simulink model "gm_uz_pmsm_model_3ph_dq_vnl"  (R2021b)
settings: Solver=FixedStepAuto  StartTime=0.0  StopTime=0.5  RelTol=1e-3
PreLoadFcn:
  | uz_pmsm_model_init_parameter
undefined symbols (not defined in the file or in its folder): friction_coefficient, inertia, k_i_d, k_p_d, k_p_q, L_d, L_q, polepair, psi_pm, R_1, setpoint_step, simulate_mechanical, simulate_open_loop, static_friction_torque, ts, ts_regler
libraries: hdlmdlgenlib x69, dspsigops x18, simulink x12, slpidlib x2
(part 2 of 2)

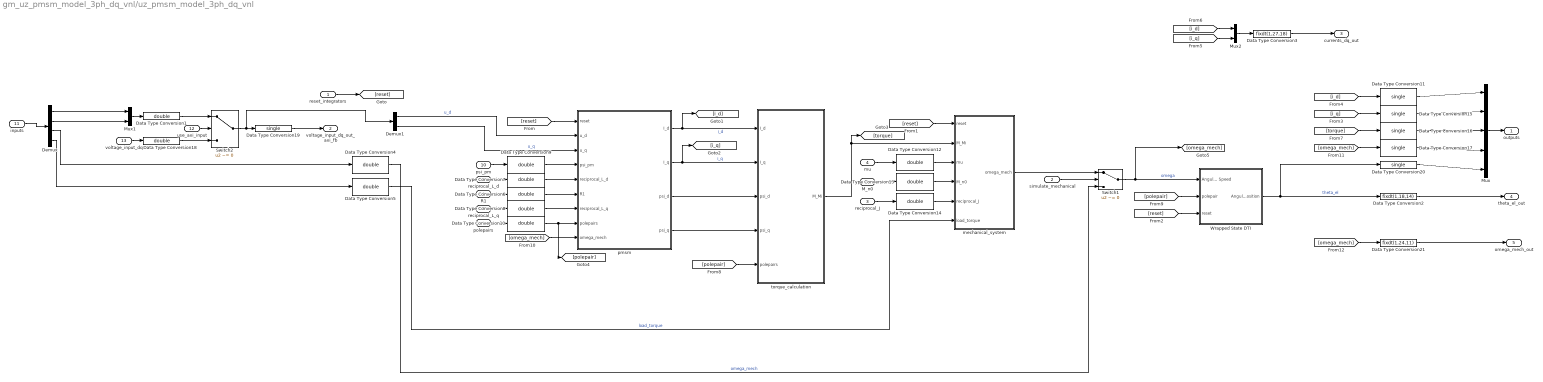
== system gm_uz_pmsm_model_3ph_dq_vnl/uz_pmsm_model_3ph_dq_vnl ==
  reset_integrators : Inport
  simulate_mechanical : Inport  Port=2
  reciprocal_J : Inport  Port=3
  mu : Inport  Port=4
  M_n0 : Inport  Port=5
  reciprocal_L_d : Inport  Port=6
  reciprocal_L_q : Inport  Port=7
  R1 : Inport  Port=8
  polepairs : Inport  Port=9
  psi_pm : Inport  Port=10
  inputs : Inport  Port=11
  use_axi_input : Inport  Port=12
  voltage_input_dq : Inport  Port=13
  Data Type Conversion{1,4..10,12..14,18} (12 alike) : DataTypeConversion  OutDataTypeStr=double  RndMeth=Nearest
  Data Type Conversion{11,15..17,19..20} (6 alike) : DataTypeConversion  OutDataTypeStr=single  RndMeth=Nearest
  Data Type Conversion2 : DataTypeConversion  OutDataTypeStr=fixdt(1,18,14)  RndMeth=Nearest
  Data Type Conversion21 : DataTypeConversion  OutDataTypeStr=fixdt(1,24,11)  RndMeth=Nearest
  Data Type Conversion3 : DataTypeConversion  OutDataTypeStr=fixdt(1,27,18)  RndMeth=Nearest
  Demux : Demux
  Demux1 : Demux  Outputs=2
  Mux : Mux  Inputs=5
  Mux1 : Mux  Inputs=2
  Mux2 : Mux  Inputs=2
  Switch1 : Switch  Criteria=u2 ~= 0
  Switch2 : Switch  Criteria=u2 ~= 0
  Wrapped State DTI : Subsystem
  mechanical_system : Subsystem
  pmsm : Subsystem
  torque_calculation : Subsystem
  outputs : Outport
  voltage_input_dq_out_axi_fb : Outport  Port=2
  currents_dq_out : Outport  Port=3
  theta_el_out : Outport  Port=4
  omega_mech_out : Outport  Port=5
  wires:
  [omega_mech] -> Data Type Conversion21/1
  Data Type Conversion21/1 -> omega_mech_out/1
  Data Type Conversion18/1 -> Switch2/3
  Data Type Conversion1/1 -> Switch2/1
  [omega_mech] -> Data Type Conversion17/1
  [omega_mech] -> pmsm/9(omega_mech)
  [polepair] -> Wrapped State DTI/2(polepair)
  [polepair] -> torque_calculation/5(polepairs)
  [torque] -> Data Type Conversion16/1
  [i_q] -> Mux2/2
  [i_d] -> Mux2/1
  [i_d] -> Data Type Conversion11/1
  [i_q] -> Data Type Conversion15/1
  pmsm/1(I_d) -> [i_d], torque_calculation/1(I_d)  "i_d"
  [reset] -> Wrapped State DTI/3(reset)
  [reset] -> mechanical_system/1(reset)
  [reset] -> pmsm/1(reset)
  reset_integrators/1 -> [reset]
  Data Type Conversion20/1 -> Mux/5
  Data Type Conversion2/1 -> theta_el_out/1
  Wrapped State DTI/1(Angular Position) -> Data Type Conversion20/1, Data Type Conversion2/1  "theta_el"
  Mux2/1 -> Data Type Conversion3/1
  Data Type Conversion3/1 -> currents_dq_out/1
  Demux/2 -> Mux1/2
  Demux/1 -> Mux1/1
  use_axi_input/1 -> Switch2/2
  Mux1/1 -> Data Type Conversion1/1
  Switch2/1 -> Data Type Conversion19/1, Demux1/1
  voltage_input_dq/1 -> Data Type Conversion18/1
  Data Type Conversion19/1 -> voltage_input_dq_out_axi_fb/1
  Mux/1 -> outputs/1
  inputs/1 -> Demux/1
  Demux/4 -> Data Type Conversion5/1
  Demux/3 -> Data Type Conversion4/1
  Data Type Conversion11/1 -> Mux/1
  Data Type Conversion15/1 -> Mux/2
  Data Type Conversion16/1 -> Mux/3
  Data Type Conversion17/1 -> Mux/4
  pmsm/2(I_q) -> torque_calculation/2(I_q), [i_q]  "i_q"
  mechanical_system/1(omega_mech) -> Switch1/1
  Demux1/2 -> pmsm/3(u_q)  "u_q"
  polepairs/1 -> Data Type Conversion10/1
  reciprocal_L_q/1 -> Data Type Conversion8/1
  Data Type Conversion8/1 -> pmsm/7(reciprocal_L_q)
  reciprocal_L_d/1 -> Data Type Conversion7/1
  Data Type Conversion13/1 -> mechanical_system/4(M_n0)
  psi_pm/1 -> Data Type Conversion9/1
  mu/1 -> Data Type Conversion12/1
  torque_calculation/1(M_Mi) -> mechanical_system/2(M_Mi), [torque]
  Data Type Conversion14/1 -> mechanical_system/5(reciprocal_J)
  M_n0/1 -> Data Type Conversion13/1
  simulate_mechanical/1 -> Switch1/2
  Data Type Conversion12/1 -> mechanical_system/3(mu)
  Demux1/1 -> pmsm/2(u_d)  "u_d"
  Data Type Conversion10/1 -> pmsm/8(polepairs), [polepair]
  pmsm/4(psi_q) -> torque_calculation/4(psi_q)
  Data Type Conversion6/1 -> pmsm/6(R1)
  R1/1 -> Data Type Conversion6/1
  Data Type Conversion9/1 -> pmsm/4(psi_pm)
  Switch1/1 -> [omega_mech], Wrapped State DTI/1(Angular Speed)  "omega"
  Data Type Conversion7/1 -> pmsm/5(reciprocal_L_d)
  Data Type Conversion5/1 -> mechanical_system/6(load_torque)  "load_torque"
  pmsm/3(psi_d) -> torque_calculation/3(psi_d)
  reciprocal_J/1 -> Data Type Conversion14/1
  Data Type Conversion4/1 -> Switch1/3  "omega_mech"

== system gm_uz_pmsm_model_3ph_dq_vnl/Compare/Assert_currents_dq_out ==
  cosim : Inport
  dut : Inport  Port=2
  AssertEq : Assertion  StopWhenAssertionFail=off
  Compare To Zero : simulink/Logic and Bit Operations/Compare To Zero  relop===  OutDataTypeStr=boolean
  Constant1 : Constant  Value=0  OutDataTypeStr=Inherit: Inherit via back propagation  SampleTime=-1
  Counter : simulink/Sources/Counter Free-Running  NumBits=32  tsamp=-1
  IgnoreCycles : Constant  Value=2  OutDataTypeStr=Inherit: Inherit via back propagation  SampleTime=-1
  Relational Operator : RelationalOperator  Operator=<  OutDataTypeStr=boolean  RndMeth=Nearest
  Relational Operator1 : RelationalOperator  Operator===  OutDataTypeStr=boolean  RndMeth=Nearest
  Switch : Switch  Criteria=u2 ~= 0
  Switch1 : Switch  Criteria=u2 ~= 0
  compare: currents_dq_out : Scope  NumInputPorts=3
  wires:
  Compare To Zero/1 -> compare: currents_dq_out/3
  Relational Operator1/1 -> Compare To Zero/1, AssertEq/1  "err"
  Switch1/1 -> compare: currents_dq_out/1, Relational Operator1/1
  Switch/1 -> compare: currents_dq_out/2, Relational Operator1/2
  Constant1/1 -> Switch/1, Switch1/1
  Relational Operator/1 -> Switch/2, Switch1/2
  cosim/1 -> Switch1/3  "cosim"
  dut/1 -> Switch/3  "dut ref"
  Counter/1 -> Relational Operator/1
  IgnoreCycles/1 -> Relational Operator/2

== system gm_uz_pmsm_model_3ph_dq_vnl/Compare/Assert_omega_mech_out ==
  cosim : Inport
  dut : Inport  Port=2
  AssertEq : Assertion  StopWhenAssertionFail=off
  Compare To Zero : simulink/Logic and Bit Operations/Compare To Zero  relop===  OutDataTypeStr=boolean
  Constant1 : Constant  Value=0  OutDataTypeStr=Inherit: Inherit via back propagation  SampleTime=-1
  Counter : simulink/Sources/Counter Free-Running  NumBits=32  tsamp=-1
  IgnoreCycles : Constant  Value=2  OutDataTypeStr=Inherit: Inherit via back propagation  SampleTime=-1
  Relational Operator : RelationalOperator  Operator=<  OutDataTypeStr=boolean  RndMeth=Nearest
  Relational Operator1 : RelationalOperator  Operator===  OutDataTypeStr=boolean  RndMeth=Nearest
  Switch : Switch  Criteria=u2 ~= 0
  Switch1 : Switch  Criteria=u2 ~= 0
  compare: omega_mech_out : Scope  NumInputPorts=3
  wires:
  Compare To Zero/1 -> compare: omega_mech_out/3
  Relational Operator1/1 -> Compare To Zero/1, AssertEq/1  "err"
  Switch1/1 -> compare: omega_mech_out/1, Relational Operator1/1
  Switch/1 -> compare: omega_mech_out/2, Relational Operator1/2
  Constant1/1 -> Switch/1, Switch1/1
  Relational Operator/1 -> Switch/2, Switch1/2
  cosim/1 -> Switch1/3  "cosim"
  dut/1 -> Switch/3  "dut ref"
  Counter/1 -> Relational Operator/1
  IgnoreCycles/1 -> Relational Operator/2

== system gm_uz_pmsm_model_3ph_dq_vnl/Compare/Assert_outputs ==
  cosim : Inport
  dut : Inport  Port=2
  AssertEq : Assertion  StopWhenAssertionFail=off
  Compare To Zero : simulink/Logic and Bit Operations/Compare To Zero  relop===  OutDataTypeStr=boolean
  Constant1 : Constant  Value=0  OutDataTypeStr=Inherit: Inherit via back propagation  SampleTime=-1
  Counter : simulink/Sources/Counter Free-Running  NumBits=32  tsamp=-1
  IgnoreCycles : Constant  Value=2  OutDataTypeStr=Inherit: Inherit via back propagation  SampleTime=-1
  RelErrCheck : Subsystem
  Relational Operator : RelationalOperator  Operator=<  OutDataTypeStr=boolean  RndMeth=Nearest
  Switch : Switch  Criteria=u2 ~= 0
  Switch1 : Switch  Criteria=u2 ~= 0
  compare: outputs : Scope  NumInputPorts=3
  wires:
  IgnoreCycles/1 -> Relational Operator/2
  Counter/1 -> Relational Operator/1
  dut/1 -> Switch/3  "dut ref"
  cosim/1 -> Switch1/3  "cosim"
  Relational Operator/1 -> Switch1/2, Switch/2
  Constant1/1 -> Switch1/1, Switch/1
  Switch/1 -> compare: outputs/2, RelErrCheck/2(In2)
  Switch1/1 -> compare: outputs/1, RelErrCheck/1(In1)
  RelErrCheck/1(Out1) -> AssertEq/1, Compare To Zero/1  "err"
  Compare To Zero/1 -> compare: outputs/3

== system gm_uz_pmsm_model_3ph_dq_vnl/Compare/Assert_theta_el_out ==
  cosim : Inport
  dut : Inport  Port=2
  AssertEq : Assertion  StopWhenAssertionFail=off
  Compare To Zero : simulink/Logic and Bit Operations/Compare To Zero  relop===  OutDataTypeStr=boolean
  Constant1 : Constant  Value=0  OutDataTypeStr=Inherit: Inherit via back propagation  SampleTime=-1
  Counter : simulink/Sources/Counter Free-Running  NumBits=32  tsamp=-1
  IgnoreCycles : Constant  Value=2  OutDataTypeStr=Inherit: Inherit via back propagation  SampleTime=-1
  Relational Operator : RelationalOperator  Operator=<  OutDataTypeStr=boolean  RndMeth=Nearest
  Relational Operator1 : RelationalOperator  Operator===  OutDataTypeStr=boolean  RndMeth=Nearest
  Switch : Switch  Criteria=u2 ~= 0
  Switch1 : Switch  Criteria=u2 ~= 0
  compare: theta_el_out : Scope  NumInputPorts=3
  wires:
  Compare To Zero/1 -> compare: theta_el_out/3
  Relational Operator1/1 -> Compare To Zero/1, AssertEq/1  "err"
  Switch1/1 -> compare: theta_el_out/1, Relational Operator1/1
  Switch/1 -> compare: theta_el_out/2, Relational Operator1/2
  Constant1/1 -> Switch/1, Switch1/1
  Relational Operator/1 -> Switch/2, Switch1/2
  cosim/1 -> Switch1/3  "cosim"
  dut/1 -> Switch/3  "dut ref"
  Counter/1 -> Relational Operator/1
  IgnoreCycles/1 -> Relational Operator/2

== system gm_uz_pmsm_model_3ph_dq_vnl/Compare/Assert_voltage_input_dq_out_axi_fb ==
  cosim : Inport
  dut : Inport  Port=2
  AssertEq : Assertion  StopWhenAssertionFail=off
  Compare To Zero : simulink/Logic and Bit Operations/Compare To Zero  relop===  OutDataTypeStr=boolean
  Constant1 : Constant  Value=0  OutDataTypeStr=Inherit: Inherit via back propagation  SampleTime=-1
  Counter : simulink/Sources/Counter Free-Running  NumBits=32  tsamp=-1
  IgnoreCycles : Constant  Value=2  OutDataTypeStr=Inherit: Inherit via back propagation  SampleTime=-1
  RelErrCheck : Subsystem
  Relational Operator : RelationalOperator  Operator=<  OutDataTypeStr=boolean  RndMeth=Nearest
  Switch : Switch  Criteria=u2 ~= 0
  Switch1 : Switch  Criteria=u2 ~= 0
  compare: voltage_input_dq_out_axi_fb : Scope  NumInputPorts=3
  wires:
  IgnoreCycles/1 -> Relational Operator/2
  Counter/1 -> Relational Operator/1
  dut/1 -> Switch/3  "dut ref"
  cosim/1 -> Switch1/3  "cosim"
  Relational Operator/1 -> Switch1/2, Switch/2
  Constant1/1 -> Switch1/1, Switch/1
  Switch/1 -> compare: voltage_input_dq_out_axi_fb/2, RelErrCheck/2(In2)
  Switch1/1 -> compare: voltage_input_dq_out_axi_fb/1, RelErrCheck/1(In1)
  RelErrCheck/1(Out1) -> AssertEq/1, Compare To Zero/1  "err"
  Compare To Zero/1 -> compare: voltage_input_dq_out_axi_fb/3

== system gm_uz_pmsm_model_3ph_dq_vnl/Compare/CleanupScopes ==

== system gm_uz_pmsm_model_3ph_dq_vnl/Compare/Enable ==

== system gm_uz_pmsm_model_3ph_dq_vnl/FOC_controller/decoupling ==
  i_d : Inport
  i_q : Inport  Port=2
  omega_m : Inport  Port=3
  Constant1 : Constant  Value=psi_pm  SampleTime=-1
  Gain : Gain  Gain=L_q
  Gain1 : Gain  Gain=L_d
  Gain2 : Gain  Gain=polepair
  Product : Product
  Product1 : Product
  Sum6 : Sum  Inputs=|++
  u_d : Outport
  u_q : Outport  Port=2
  wires:
  Gain/1 -> Product/1
  Gain2/1 -> Product1/2, Product/2
  Product1/1 -> u_q/1
  i_d/1 -> Gain1/1
  Product/1 -> u_d/1
  Gain1/1 -> Sum6/1
  i_q/1 -> Gain/1
  Constant1/1 -> Sum6/2
  Sum6/1 -> Product1/1
  omega_m/1 -> Gain2/1

== system gm_uz_pmsm_model_3ph_dq_vnl/uz_pmsm_model_3ph_dq/Abs ==
  In1 : Inport
  Abs : Abs  SampleTime=1e-08  OutDataTypeStr=double
  Out1 : Outport
  wires:
  Abs/1 -> Out1/1
  In1/1 -> Abs/1

== system gm_uz_pmsm_model_3ph_dq_vnl/uz_pmsm_model_3ph_dq/Compare To Constant1_relop ==
  In1 : Inport
  In2 : Inport  Port=2
  Compare To Constant1_relop : RelationalOperator  Operator=<  OutDataTypeStr=boolean  SampleTime=1e-08  RndMeth=Nearest  InputSameDT=on
  Compare To Constant1_relop_pd1 : Delay  DelayLength=1
  Out1 : Outport
  wires:
  Compare To Constant1_relop_pd1/1 -> Out1/1
  Compare To Constant1_relop/1 -> Compare To Constant1_relop_pd1/1
  In2/1 -> Compare To Constant1_relop/2
  In1/1 -> Compare To Constant1_relop/1

== system gm_uz_pmsm_model_3ph_dq_vnl/uz_pmsm_model_3ph_dq/Compare To Constant_relop ==
  In1 : Inport
  In2 : Inport  Port=2
  Compare To Constant_relop : RelationalOperator  OutDataTypeStr=boolean  SampleTime=1e-08  RndMeth=Nearest  InputSameDT=on
  Compare To Constant_relop_pd1 : Delay  DelayLength=1
  Out1 : Outport
  wires:
  Compare To Constant_relop_pd1/1 -> Out1/1
  Compare To Constant_relop/1 -> Compare To Constant_relop_pd1/1
  In2/1 -> Compare To Constant_relop/2
  In1/1 -> Compare To Constant_relop/1

== system gm_uz_pmsm_model_3ph_dq_vnl/uz_pmsm_model_3ph_dq/Data Type Conversion1 ==
  In1 : Inport
  Data Type Conversion1 : DataTypeConversion  OutDataTypeStr=double  RndMeth=Nearest  SampleTime=1e-08
  Data Type Conversion1_pd1 : Delay  DelayLength=3
  Out1 : Outport
  wires:
  Data Type Conversion1_pd1/1 -> Out1/1
  Data Type Conversion1/1 -> Data Type Conversion1_pd1/1
  In1/1 -> Data Type Conversion1/1

== system gm_uz_pmsm_model_3ph_dq_vnl/uz_pmsm_model_3ph_dq/Data Type Conversion10 ==
  In1 : Inport
  Data Type Conversion10 : DataTypeConversion  OutDataTypeStr=double  RndMeth=Nearest  SampleTime=1e-08
  Data Type Conversion10_pd1 : Delay  DelayLength=3
  Out1 : Outport
  wires:
  Data Type Conversion10_pd1/1 -> Out1/1
  Data Type Conversion10/1 -> Data Type Conversion10_pd1/1
  In1/1 -> Data Type Conversion10/1

== system gm_uz_pmsm_model_3ph_dq_vnl/uz_pmsm_model_3ph_dq/Data Type Conversion11 ==
  In1 : Inport
  Data Type Conversion11 : DataTypeConversion  OutDataTypeStr=single  RndMeth=Nearest  SampleTime=1e-08
  Data Type Conversion11_pd1 : Delay  DelayLength=3
  Out1 : Outport
  wires:
  Data Type Conversion11_pd1/1 -> Out1/1
  Data Type Conversion11/1 -> Data Type Conversion11_pd1/1
  In1/1 -> Data Type Conversion11/1

== system gm_uz_pmsm_model_3ph_dq_vnl/uz_pmsm_model_3ph_dq/Data Type Conversion12 ==
  In1 : Inport
  Data Type Conversion12 : DataTypeConversion  OutDataTypeStr=double  RndMeth=Nearest  SampleTime=1e-08
  Data Type Conversion12_pd1 : Delay  DelayLength=3
  Out1 : Outport
  wires:
  Data Type Conversion12_pd1/1 -> Out1/1
  Data Type Conversion12/1 -> Data Type Conversion12_pd1/1
  In1/1 -> Data Type Conversion12/1

== system gm_uz_pmsm_model_3ph_dq_vnl/uz_pmsm_model_3ph_dq/Data Type Conversion13 ==
  In1 : Inport
  Data Type Conversion13 : DataTypeConversion  OutDataTypeStr=double  RndMeth=Nearest  SampleTime=1e-08
  Data Type Conversion13_pd1 : Delay  DelayLength=3
  Out1 : Outport
  wires:
  Data Type Conversion13_pd1/1 -> Out1/1
  Data Type Conversion13/1 -> Data Type Conversion13_pd1/1
  In1/1 -> Data Type Conversion13/1

== system gm_uz_pmsm_model_3ph_dq_vnl/uz_pmsm_model_3ph_dq/Data Type Conversion14 ==
  In1 : Inport
  Data Type Conversion14 : DataTypeConversion  OutDataTypeStr=double  RndMeth=Nearest  SampleTime=1e-08
  Data Type Conversion14_pd1 : Delay  DelayLength=3
  Out1 : Outport
  wires:
  Data Type Conversion14_pd1/1 -> Out1/1
  Data Type Conversion14/1 -> Data Type Conversion14_pd1/1
  In1/1 -> Data Type Conversion14/1

== system gm_uz_pmsm_model_3ph_dq_vnl/uz_pmsm_model_3ph_dq/Data Type Conversion15 ==
  In1 : Inport
  Data Type Conversion15 : DataTypeConversion  OutDataTypeStr=single  RndMeth=Nearest  SampleTime=1e-08
  Data Type Conversion15_pd1 : Delay  DelayLength=3
  Out1 : Outport
  wires:
  Data Type Conversion15_pd1/1 -> Out1/1
  Data Type Conversion15/1 -> Data Type Conversion15_pd1/1
  In1/1 -> Data Type Conversion15/1

== system gm_uz_pmsm_model_3ph_dq_vnl/uz_pmsm_model_3ph_dq/Data Type Conversion16 ==
  In1 : Inport
  Data Type Conversion16 : DataTypeConversion  OutDataTypeStr=single  RndMeth=Nearest  SampleTime=1e-08
  Data Type Conversion16_pd1 : Delay  DelayLength=3
  Out1 : Outport
  wires:
  Data Type Conversion16_pd1/1 -> Out1/1
  Data Type Conversion16/1 -> Data Type Conversion16_pd1/1
  In1/1 -> Data Type Conversion16/1

== system gm_uz_pmsm_model_3ph_dq_vnl/uz_pmsm_model_3ph_dq/Data Type Conversion17 ==
  In1 : Inport
  Data Type Conversion17 : DataTypeConversion  OutDataTypeStr=single  RndMeth=Nearest  SampleTime=1e-08
  Data Type Conversion17_pd1 : Delay  DelayLength=3
  Out1 : Outport
  wires:
  Data Type Conversion17_pd1/1 -> Out1/1
  Data Type Conversion17/1 -> Data Type Conversion17_pd1/1
  In1/1 -> Data Type Conversion17/1

== system gm_uz_pmsm_model_3ph_dq_vnl/uz_pmsm_model_3ph_dq/Data Type Conversion18 ==
  In1 : Inport
  Data Type Conversion18 : DataTypeConversion  OutDataTypeStr=double  RndMeth=Nearest  SampleTime=1e-08
  Data Type Conversion18_pd1 : Delay  DelayLength=3
  Out1 : Outport
  wires:
  Data Type Conversion18_pd1/1 -> Out1/1
  Data Type Conversion18/1 -> Data Type Conversion18_pd1/1
  In1/1 -> Data Type Conversion18/1

== system gm_uz_pmsm_model_3ph_dq_vnl/uz_pmsm_model_3ph_dq/Data Type Conversion19 ==
  In1 : Inport
  Data Type Conversion19 : DataTypeConversion  OutDataTypeStr=single  RndMeth=Nearest  SampleTime=1e-08
  Data Type Conversion19_pd1 : Delay  DelayLength=3
  Out1 : Outport
  wires:
  Data Type Conversion19_pd1/1 -> Out1/1
  Data Type Conversion19/1 -> Data Type Conversion19_pd1/1
  In1/1 -> Data Type Conversion19/1

== system gm_uz_pmsm_model_3ph_dq_vnl/uz_pmsm_model_3ph_dq/Data Type Conversion2 ==
  In1 : Inport
  Data Type Conversion2 : DataTypeConversion  OutDataTypeStr=fixdt(1, 18, 14)  RndMeth=Nearest  SampleTime=1e-08
  Data Type Conversion2_pd1 : Delay  DelayLength=3
  Out1 : Outport
  wires:
  Data Type Conversion2_pd1/1 -> Out1/1
  Data Type Conversion2/1 -> Data Type Conversion2_pd1/1
  In1/1 -> Data Type Conversion2/1

== system gm_uz_pmsm_model_3ph_dq_vnl/uz_pmsm_model_3ph_dq/Data Type Conversion20 ==
  In1 : Inport
  Data Type Conversion20 : DataTypeConversion  OutDataTypeStr=single  RndMeth=Nearest  SampleTime=1e-08
  Data Type Conversion20_pd1 : Delay  DelayLength=3
  Out1 : Outport
  wires:
  Data Type Conversion20_pd1/1 -> Out1/1
  Data Type Conversion20/1 -> Data Type Conversion20_pd1/1
  In1/1 -> Data Type Conversion20/1

== system gm_uz_pmsm_model_3ph_dq_vnl/uz_pmsm_model_3ph_dq/Data Type Conversion21 ==
  In1 : Inport
  Data Type Conversion21 : DataTypeConversion  OutDataTypeStr=fixdt(1, 24, 11)  RndMeth=Nearest  SampleTime=1e-08
  Data Type Conversion21_pd1 : Delay  DelayLength=3
  Out1 : Outport
  wires:
  Data Type Conversion21_pd1/1 -> Out1/1
  Data Type Conversion21/1 -> Data Type Conversion21_pd1/1
  In1/1 -> Data Type Conversion21/1

== system gm_uz_pmsm_model_3ph_dq_vnl/uz_pmsm_model_3ph_dq/Data Type Conversion3 ==
  In1 : Inport
  Data Type Conversion3 : DataTypeConversion  OutDataTypeStr=fixdt(1, 27, 18)  RndMeth=Nearest  SampleTime=1e-08
  Data Type Conversion3_pd1 : Delay  DelayLength=3
  Out1 : Outport
  wires:
  Data Type Conversion3_pd1/1 -> Out1/1
  Data Type Conversion3/1 -> Data Type Conversion3_pd1/1
  In1/1 -> Data Type Conversion3/1

== system gm_uz_pmsm_model_3ph_dq_vnl/uz_pmsm_model_3ph_dq/Data Type Conversion4 ==
  In1 : Inport
  Data Type Conversion4 : DataTypeConversion  OutDataTypeStr=double  RndMeth=Nearest  SampleTime=1e-08
  Data Type Conversion4_pd1 : Delay  DelayLength=3
  Out1 : Outport
  wires:
  Data Type Conversion4_pd1/1 -> Out1/1
  Data Type Conversion4/1 -> Data Type Conversion4_pd1/1
  In1/1 -> Data Type Conversion4/1

== system gm_uz_pmsm_model_3ph_dq_vnl/uz_pmsm_model_3ph_dq/Data Type Conversion5 ==
  In1 : Inport
  Data Type Conversion5 : DataTypeConversion  OutDataTypeStr=double  RndMeth=Nearest  SampleTime=1e-08
  Data Type Conversion5_pd1 : Delay  DelayLength=3
  Out1 : Outport
  wires:
  Data Type Conversion5_pd1/1 -> Out1/1
  Data Type Conversion5/1 -> Data Type Conversion5_pd1/1
  In1/1 -> Data Type Conversion5/1

== system gm_uz_pmsm_model_3ph_dq_vnl/uz_pmsm_model_3ph_dq/Data Type Conversion6 ==
  In1 : Inport
  Data Type Conversion6 : DataTypeConversion  OutDataTypeStr=double  RndMeth=Nearest  SampleTime=1e-08
  Data Type Conversion6_pd1 : Delay  DelayLength=3
  Out1 : Outport
  wires:
  Data Type Conversion6_pd1/1 -> Out1/1
  Data Type Conversion6/1 -> Data Type Conversion6_pd1/1
  In1/1 -> Data Type Conversion6/1

== system gm_uz_pmsm_model_3ph_dq_vnl/uz_pmsm_model_3ph_dq/Data Type Conversion7 ==
  In1 : Inport
  Data Type Conversion7 : DataTypeConversion  OutDataTypeStr=double  RndMeth=Nearest  SampleTime=1e-08
  Data Type Conversion7_pd1 : Delay  DelayLength=3
  Out1 : Outport
  wires:
  Data Type Conversion7_pd1/1 -> Out1/1
  Data Type Conversion7/1 -> Data Type Conversion7_pd1/1
  In1/1 -> Data Type Conversion7/1

== system gm_uz_pmsm_model_3ph_dq_vnl/uz_pmsm_model_3ph_dq/Data Type Conversion8 ==
  In1 : Inport
  Data Type Conversion8 : DataTypeConversion  OutDataTypeStr=double  RndMeth=Nearest  SampleTime=1e-08
  Data Type Conversion8_pd1 : Delay  DelayLength=3
  Out1 : Outport
  wires:
  Data Type Conversion8_pd1/1 -> Out1/1
  Data Type Conversion8/1 -> Data Type Conversion8_pd1/1
  In1/1 -> Data Type Conversion8/1

== system gm_uz_pmsm_model_3ph_dq_vnl/uz_pmsm_model_3ph_dq/Data Type Conversion9 ==
  In1 : Inport
  Data Type Conversion9 : DataTypeConversion  OutDataTypeStr=double  RndMeth=Nearest  SampleTime=1e-08
  Data Type Conversion9_pd1 : Delay  DelayLength=3
  Out1 : Outport
  wires:
  Data Type Conversion9_pd1/1 -> Out1/1
  Data Type Conversion9/1 -> Data Type Conversion9_pd1/1
  In1/1 -> Data Type Conversion9/1

== system gm_uz_pmsm_model_3ph_dq_vnl/uz_pmsm_model_3ph_dq/Factor ==
  In1 : Inport
  In2 : Inport  Port=2
  Factor : Product  Inputs=**  OutDataTypeStr=double  SampleTime=1e-08
  Factor_pd1 : Delay  DelayLength=6
  Out1 : Outport
  wires:
  Factor_pd1/1 -> Out1/1
  Factor/1 -> Factor_pd1/1
  In2/1 -> Factor/2
  In1/1 -> Factor/1

== system gm_uz_pmsm_model_3ph_dq_vnl/uz_pmsm_model_3ph_dq/Gain ==
  In1 : Inport
  In2 : Inport  Port=2
  Gain : Product  Inputs=**  OutDataTypeStr=double  SampleTime=1e-08
  Gain_pd1 : Delay  DelayLength=6
  Out1 : Outport
  wires:
  Gain_pd1/1 -> Out1/1
  Gain/1 -> Gain_pd1/1
  In2/1 -> Gain/2
  In1/1 -> Gain/1

== system gm_uz_pmsm_model_3ph_dq_vnl/uz_pmsm_model_3ph_dq/Gain1 ==
  In1 : Inport
  In2 : Inport  Port=2
  Gain1 : Product  Inputs=**  OutDataTypeStr=double  SampleTime=1e-08
  Gain1_pd1 : Delay  DelayLength=6
  Out1 : Outport
  wires:
  Gain1_pd1/1 -> Out1/1
  Gain1/1 -> Gain1_pd1/1
  In2/1 -> Gain1/2
  In1/1 -> Gain1/1

== system gm_uz_pmsm_model_3ph_dq_vnl/uz_pmsm_model_3ph_dq/Gain2 ==
  In1 : Inport
  In2 : Inport  Port=2
  Gain2 : Product  Inputs=**  OutDataTypeStr=double  SampleTime=1e-08
  Gain2_pd1 : Delay  DelayLength=6
  Out1 : Outport
  wires:
  Gain2_pd1/1 -> Out1/1
  Gain2/1 -> Gain2_pd1/1
  In2/1 -> Gain2/2
  In1/1 -> Gain2/1

== system gm_uz_pmsm_model_3ph_dq_vnl/uz_pmsm_model_3ph_dq/Gain3 ==
  In1 : Inport
  In2 : Inport  Port=2
  Gain3 : Product  Inputs=**  OutDataTypeStr=double  SampleTime=1e-08
  Gain3_pd1 : Delay  DelayLength=6
  Out1 : Outport
  wires:
  Gain3_pd1/1 -> Out1/1
  Gain3/1 -> Gain3_pd1/1
  In2/1 -> Gain3/2
  In1/1 -> Gain3/1

== system gm_uz_pmsm_model_3ph_dq_vnl/uz_pmsm_model_3ph_dq/Product ==
  In1 : Inport
  In2 : Inport  Port=2
  Product : Product  Inputs=**  OutDataTypeStr=double  SampleTime=1e-08
  Product_pd1 : Delay  DelayLength=6
  Out1 : Outport
  wires:
  Product_pd1/1 -> Out1/1
  Product/1 -> Product_pd1/1
  In2/1 -> Product/2
  In1/1 -> Product/1

== system gm_uz_pmsm_model_3ph_dq_vnl/uz_pmsm_model_3ph_dq/Product1 ==
  In1 : Inport
  In2 : Inport  Port=2
  Product1 : Product  Inputs=**  OutDataTypeStr=double  SampleTime=1e-08
  Product1_pd1 : Delay  DelayLength=6
  Out1 : Outport
  wires:
  Product1_pd1/1 -> Out1/1
  Product1/1 -> Product1_pd1/1
  In2/1 -> Product1/2
  In1/1 -> Product1/1

== system gm_uz_pmsm_model_3ph_dq_vnl/uz_pmsm_model_3ph_dq/Product10 ==
  In1 : Inport
  In2 : Inport  Port=2
  Product10 : Product  Inputs=**  OutDataTypeStr=double  SampleTime=1e-08
  Product10_pd1 : Delay  DelayLength=6
  Out1 : Outport
  wires:
  Product10_pd1/1 -> Out1/1
  Product10/1 -> Product10_pd1/1
  In2/1 -> Product10/2
  In1/1 -> Product10/1

== system gm_uz_pmsm_model_3ph_dq_vnl/uz_pmsm_model_3ph_dq/Product11 ==
  In1 : Inport
  In2 : Inport  Port=2
  Product11 : Product  Inputs=**  OutDataTypeStr=double  SampleTime=1e-08
  Product11_pd1 : Delay  DelayLength=6
  Out1 : Outport
  wires:
  Product11_pd1/1 -> Out1/1
  Product11/1 -> Product11_pd1/1
  In2/1 -> Product11/2
  In1/1 -> Product11/1

== system gm_uz_pmsm_model_3ph_dq_vnl/uz_pmsm_model_3ph_dq/Product12 ==
  In1 : Inport
  In2 : Inport  Port=2
  Product12 : Product  Inputs=**  OutDataTypeStr=double  SampleTime=1e-08
  Product12_pd1 : Delay  DelayLength=6
  Out1 : Outport
  wires:
  Product12_pd1/1 -> Out1/1
  Product12/1 -> Product12_pd1/1
  In2/1 -> Product12/2
  In1/1 -> Product12/1

== system gm_uz_pmsm_model_3ph_dq_vnl/uz_pmsm_model_3ph_dq/Product2 ==
  In1 : Inport
  In2 : Inport  Port=2
  Product2 : Product  Inputs=**  OutDataTypeStr=double  SampleTime=1e-08
  Product2_pd1 : Delay  DelayLength=6
  Out1 : Outport
  wires:
  Product2_pd1/1 -> Out1/1
  Product2/1 -> Product2_pd1/1
  In2/1 -> Product2/2
  In1/1 -> Product2/1

== system gm_uz_pmsm_model_3ph_dq_vnl/uz_pmsm_model_3ph_dq/Product3 ==
  In1 : Inport
  In2 : Inport  Port=2
  Product3 : Product  Inputs=**  OutDataTypeStr=double  SampleTime=1e-08
  Product3_pd1 : Delay  DelayLength=6
  Out1 : Outport
  wires:
  Product3_pd1/1 -> Out1/1
  Product3/1 -> Product3_pd1/1
  In2/1 -> Product3/2
  In1/1 -> Product3/1

== system gm_uz_pmsm_model_3ph_dq_vnl/uz_pmsm_model_3ph_dq/Product31 ==
  In1 : Inport
  In2 : Inport  Port=2
  Product31 : Product  Inputs=**  OutDataTypeStr=double  SampleTime=1e-08
  Product31_pd1 : Delay  DelayLength=6
  Out1 : Outport
  wires:
  Product31_pd1/1 -> Out1/1
  Product31/1 -> Product31_pd1/1
  In2/1 -> Product31/2
  In1/1 -> Product31/1

== system gm_uz_pmsm_model_3ph_dq_vnl/uz_pmsm_model_3ph_dq/Product4 ==
  In1 : Inport
  In2 : Inport  Port=2
  Product4 : Product  Inputs=**  OutDataTypeStr=double  SampleTime=1e-08
  Product4_pd1 : Delay  DelayLength=6
  Out1 : Outport
  wires:
  Product4_pd1/1 -> Out1/1
  Product4/1 -> Product4_pd1/1
  In2/1 -> Product4/2
  In1/1 -> Product4/1

== system gm_uz_pmsm_model_3ph_dq_vnl/uz_pmsm_model_3ph_dq/Product5 ==
  In1 : Inport
  In2 : Inport  Port=2
  Product5 : Product  Inputs=**  OutDataTypeStr=double  SampleTime=1e-08
  Product5_pd1 : Delay  DelayLength=6
  Out1 : Outport
  wires:
  Product5_pd1/1 -> Out1/1
  Product5/1 -> Product5_pd1/1
  In2/1 -> Product5/2
  In1/1 -> Product5/1

== system gm_uz_pmsm_model_3ph_dq_vnl/uz_pmsm_model_3ph_dq/Product6 ==
  In1 : Inport
  In2 : Inport  Port=2
  Product6 : Product  Inputs=**  OutDataTypeStr=double  SampleTime=1e-08
  Product6_pd1 : Delay  DelayLength=6
  Out1 : Outport
  wires:
  Product6_pd1/1 -> Out1/1
  Product6/1 -> Product6_pd1/1
  In2/1 -> Product6/2
  In1/1 -> Product6/1

== system gm_uz_pmsm_model_3ph_dq_vnl/uz_pmsm_model_3ph_dq/Product7 ==
  In1 : Inport
  In2 : Inport  Port=2
  Product7 : Product  Inputs=**  OutDataTypeStr=double  SampleTime=1e-08
  Product7_pd1 : Delay  DelayLength=6
  Out1 : Outport
  wires:
  Product7_pd1/1 -> Out1/1
  Product7/1 -> Product7_pd1/1
  In2/1 -> Product7/2
  In1/1 -> Product7/1

== system gm_uz_pmsm_model_3ph_dq_vnl/uz_pmsm_model_3ph_dq/Product8 ==
  In1 : Inport
  In2 : Inport  Port=2
  Product8 : Product  Inputs=**  OutDataTypeStr=double  SampleTime=1e-08
  Product8_pd1 : Delay  DelayLength=6
  Out1 : Outport
  wires:
  Product8_pd1/1 -> Out1/1
  Product8/1 -> Product8_pd1/1
  In2/1 -> Product8/2
  In1/1 -> Product8/1

== system gm_uz_pmsm_model_3ph_dq_vnl/uz_pmsm_model_3ph_dq/Product9 ==
  In1 : Inport
  In2 : Inport  Port=2
  Product9 : Product  Inputs=**  OutDataTypeStr=double  SampleTime=1e-08
  Product9_pd1 : Delay  DelayLength=6
  Out1 : Outport
  wires:
  Product9_pd1/1 -> Out1/1
  Product9/1 -> Product9_pd1/1
  In2/1 -> Product9/2
  In1/1 -> Product9/1

== system gm_uz_pmsm_model_3ph_dq_vnl/uz_pmsm_model_3ph_dq/Sign1 ==
  In1 : Inport
  Sign1 : Signum  SampleTime=1e-08
  Out1 : Outport
  wires:
  Sign1/1 -> Out1/1
  In1/1 -> Sign1/1

== system gm_uz_pmsm_model_3ph_dq_vnl/uz_pmsm_model_3ph_dq/Sum ==
  In1 : Inport
  In2 : Inport  Port=2
  Sum : Sum  Inputs=+-  OutDataTypeStr=double  SampleTime=1e-08
  Sum_pd1 : Delay  DelayLength=6
  Out1 : Outport
  wires:
  Sum_pd1/1 -> Out1/1
  Sum/1 -> Sum_pd1/1
  In2/1 -> Sum/2
  In1/1 -> Sum/1

== system gm_uz_pmsm_model_3ph_dq_vnl/uz_pmsm_model_3ph_dq/Sum1 ==
  In1 : Inport
  In2 : Inport  Port=2
  Sum1 : Sum  Inputs=+-  OutDataTypeStr=double  SampleTime=1e-08
  Sum1_pd1 : Delay  DelayLength=6
  Out1 : Outport
  wires:
  Sum1_pd1/1 -> Out1/1
  Sum1/1 -> Sum1_pd1/1
  In2/1 -> Sum1/2
  In1/1 -> Sum1/1

== system gm_uz_pmsm_model_3ph_dq_vnl/uz_pmsm_model_3ph_dq/Sum11 ==
  In1 : Inport
  In2 : Inport  Port=2
  Sum11 : Sum  Inputs=+-  OutDataTypeStr=double  SampleTime=1e-08
  Sum11_pd1 : Delay  DelayLength=6
  Out1 : Outport
  wires:
  Sum11_pd1/1 -> Out1/1
  Sum11/1 -> Sum11_pd1/1
  In2/1 -> Sum11/2
  In1/1 -> Sum11/1

== system gm_uz_pmsm_model_3ph_dq_vnl/uz_pmsm_model_3ph_dq/Sum1_stage2 ==
  In1 : Inport
  In2 : Inport  Port=2
  Sum1_stage2 : Sum  Inputs=+-  OutDataTypeStr=double  SampleTime=1e-08
  Sum1_stage2_pd1 : Delay  DelayLength=6
  Out1 : Outport
  wires:
  Sum1_stage2_pd1/1 -> Out1/1
  Sum1_stage2/1 -> Sum1_stage2_pd1/1
  In2/1 -> Sum1_stage2/2
  In1/1 -> Sum1_stage2/1

== system gm_uz_pmsm_model_3ph_dq_vnl/uz_pmsm_model_3ph_dq/Sum1_stage3 ==
  In1 : Inport
  In2 : Inport  Port=2
  Sum1_stage3 : Sum  Inputs=+-  OutDataTypeStr=double  SampleTime=1e-08
  Sum1_stage3_pd1 : Delay  DelayLength=6
  Out1 : Outport
  wires:
  Sum1_stage3_pd1/1 -> Out1/1
  Sum1_stage3/1 -> Sum1_stage3_pd1/1
  In2/1 -> Sum1_stage3/2
  In1/1 -> Sum1_stage3/1

== system gm_uz_pmsm_model_3ph_dq_vnl/uz_pmsm_model_3ph_dq/Sum2 ==
  In1 : Inport
  In2 : Inport  Port=2
  Sum2 : Sum  Inputs=+-  OutDataTypeStr=double  SampleTime=1e-08
  Sum2_pd1 : Delay  DelayLength=6
  Out1 : Outport
  wires:
  Sum2_pd1/1 -> Out1/1
  Sum2/1 -> Sum2_pd1/1
  In2/1 -> Sum2/2
  In1/1 -> Sum2/1

== system gm_uz_pmsm_model_3ph_dq_vnl/uz_pmsm_model_3ph_dq/Sum21 ==
  In1 : Inport
  In2 : Inport  Port=2
  Sum21 : Sum  OutDataTypeStr=double  SampleTime=1e-08
  Sum21_pd1 : Delay  DelayLength=6
  Out1 : Outport
  wires:
  Sum21_pd1/1 -> Out1/1
  Sum21/1 -> Sum21_pd1/1
  In2/1 -> Sum21/2
  In1/1 -> Sum21/1

== system gm_uz_pmsm_model_3ph_dq_vnl/uz_pmsm_model_3ph_dq/Sum3 ==
  In1 : Inport
  In2 : Inport  Port=2
  Sum3 : Sum  OutDataTypeStr=double  SampleTime=1e-08
  Sum3_pd1 : Delay  DelayLength=6
  Out1 : Outport
  wires:
  Sum3_pd1/1 -> Out1/1
  Sum3/1 -> Sum3_pd1/1
  In2/1 -> Sum3/2
  In1/1 -> Sum3/1

== system gm_uz_pmsm_model_3ph_dq_vnl/uz_pmsm_model_3ph_dq/Sum31 ==
  In1 : Inport
  In2 : Inport  Port=2
  Sum31 : Sum  OutDataTypeStr=double  SampleTime=1e-08
  Sum31_pd1 : Delay  DelayLength=6
  Out1 : Outport
  wires:
  Sum31_pd1/1 -> Out1/1
  Sum31/1 -> Sum31_pd1/1
  In2/1 -> Sum31/2
  In1/1 -> Sum31/1

== system gm_uz_pmsm_model_3ph_dq_vnl/uz_pmsm_model_3ph_dq/Sum32 ==
  In1 : Inport
  In2 : Inport  Port=2
  Sum32 : Sum  Inputs=+-  OutDataTypeStr=double  SampleTime=1e-08
  Sum32_pd1 : Delay  DelayLength=6
  Out1 : Outport
  wires:
  Sum32_pd1/1 -> Out1/1
  Sum32/1 -> Sum32_pd1/1
  In2/1 -> Sum32/2
  In1/1 -> Sum32/1

== system gm_uz_pmsm_model_3ph_dq_vnl/uz_pmsm_model_3ph_dq/Sum33 ==
  In1 : Inport
  In2 : Inport  Port=2
  Sum33 : Sum  OutDataTypeStr=double  SampleTime=1e-08
  Sum33_pd1 : Delay  DelayLength=6
  Out1 : Outport
  wires:
  Sum33_pd1/1 -> Out1/1
  Sum33/1 -> Sum33_pd1/1
  In2/1 -> Sum33/2
  In1/1 -> Sum33/1

== system gm_uz_pmsm_model_3ph_dq_vnl/uz_pmsm_model_3ph_dq/Sum4 ==
  In1 : Inport
  In2 : Inport  Port=2
  Sum4 : Sum  OutDataTypeStr=double  SampleTime=1e-08
  Sum4_pd1 : Delay  DelayLength=6
  Out1 : Outport
  wires:
  Sum4_pd1/1 -> Out1/1
  Sum4/1 -> Sum4_pd1/1
  In2/1 -> Sum4/2
  In1/1 -> Sum4/1

== system gm_uz_pmsm_model_3ph_dq_vnl/uz_pmsm_model_3ph_dq/Sum5 ==
  In1 : Inport
  In2 : Inport  Port=2
  Sum5 : Sum  OutDataTypeStr=double  SampleTime=1e-08
  Sum5_pd1 : Delay  DelayLength=6
  Out1 : Outport
  wires:
  Sum5_pd1/1 -> Out1/1
  Sum5/1 -> Sum5_pd1/1
  In2/1 -> Sum5/2
  In1/1 -> Sum5/1

== system gm_uz_pmsm_model_3ph_dq_vnl/uz_pmsm_model_3ph_dq/Sum_stage2 ==
  In1 : Inport
  In2 : Inport  Port=2
  Sum_stage2 : Sum  Inputs=+-  OutDataTypeStr=double  SampleTime=1e-08
  Sum_stage2_pd1 : Delay  DelayLength=6
  Out1 : Outport
  wires:
  Sum_stage2_pd1/1 -> Out1/1
  Sum_stage2/1 -> Sum_stage2_pd1/1
  In2/1 -> Sum_stage2/2
  In1/1 -> Sum_stage2/1

== system gm_uz_pmsm_model_3ph_dq_vnl/uz_pmsm_model_3ph_dq/Sum_stage3 ==
  In1 : Inport
  In2 : Inport  Port=2
  Sum_stage3 : Sum  OutDataTypeStr=double  SampleTime=1e-08
  Sum_stage3_pd1 : Delay  DelayLength=6
  Out1 : Outport
  wires:
  Sum_stage3_pd1/1 -> Out1/1
  Sum_stage3/1 -> Sum_stage3_pd1/1
  In2/1 -> Sum_stage3/2
  In1/1 -> Sum_stage3/1

== system gm_uz_pmsm_model_3ph_dq_vnl/uz_pmsm_model_3ph_dq_vnl/Wrapped State DTI ==
  note: https://de.mathworks.com/help/releases/R2021a/hdlcoder/ug/troubleshoot-generate-implementation-model-from-simscape-pmsm.html?searchHighlight=troubleshoot-generate-implementation-model-from-simscape-pmsm&s_tid=doc_srchtitle
  Angular Speed : Inport
  polepair : Inport  Port=2
  reset : Inport  Port=3
  Compare To Constant : simulink/Logic and Bit Operations/Compare To Constant  relop=>=  const=single(pi)  OutDataTypeStr=boolean
  Compare To Constant1 : simulink/Logic and Bit Operations/Compare To Constant  relop=<  const=single(-pi)  OutDataTypeStr=boolean
  Constant : Constant  Value=double(2*pi)  SampleTime=-1
  Delay1 : Delay  DelayLength=1  ExternalReset=Level
      settings: InputPortMap=u0,r5
  Gain : Gain  Gain=ts
  Product : Product
  Sum : Sum  Inputs=|++
  Sum1 : Sum  Inputs=|-+
  Sum2 : Sum  Inputs=|++
  Switch : Switch  Criteria=u2 > Threshold
  Switch1 : Switch  Criteria=u2 > Threshold
  Angular Position : Outport
  wires:
  polepair/1 -> Product/2
  Angular Speed/1 -> Product/1
  Product/1 -> Gain/1
  reset/1 -> Delay1/2
  Gain/1 -> Sum/2
  Sum1/1 -> Switch/1
  Sum/1 -> Switch/3, Sum1/2, Compare To Constant/1
  Compare To Constant/1 -> Switch/2
  Switch/1 -> Switch1/3, Compare To Constant1/1, Sum2/2
  Switch1/1 -> Delay1/1  "Angular Position"
  Sum2/1 -> Switch1/1
  Constant/1 -> Sum1/1, Sum2/1
  Delay1/1 -> Angular Position/1, Sum/1
  Compare To Constant1/1 -> Switch1/2

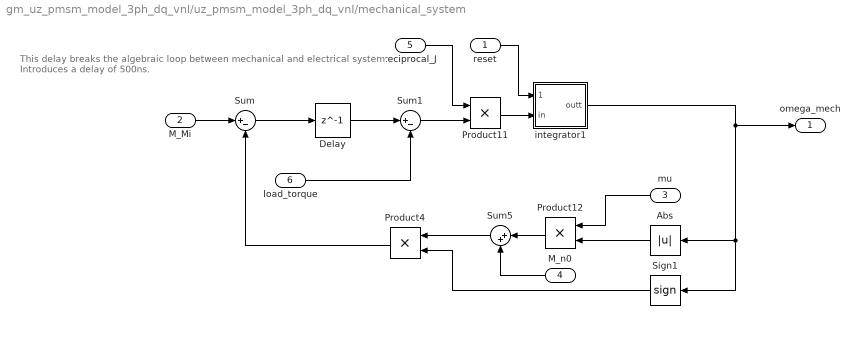
== system gm_uz_pmsm_model_3ph_dq_vnl/uz_pmsm_model_3ph_dq_vnl/mechanical_system ==
  note: This delay breaks the algebraic loop between mechanical and electrical system.
      | Introduces a delay of 500ns.
  reset : Inport
  M_Mi : Inport  Port=2
  mu : Inport  Port=3
  M_n0 : Inport  Port=4
  reciprocal_J : Inport  Port=5
  load_torque : Inport  Port=6
  Abs : Abs
  Delay : Delay  DelayLength=1
  Product11 : Product
  Product12 : Product
  Product4 : Product
  Sign1 : Signum
  Sum : Sum  Inputs=|+-
  Sum1 : Sum  Inputs=|+-
  Sum5 : Sum  Inputs=|++
  integrator1 : Subsystem
  omega_mech : Outport
  wires:
  Delay/1 -> Sum1/1
  Product4/1 -> Sum/2
  Sum/1 -> Delay/1
  load_torque/1 -> Sum1/2
  Sum1/1 -> Product11/2
  M_Mi/1 -> Sum/1
  reciprocal_J/1 -> Product11/1
  M_n0/1 -> Sum5/2
  mu/1 -> Product12/1
  Product12/1 -> Sum5/1
  reset/1 -> integrator1/1(reset)
  Abs/1 -> Product12/2
  integrator1/1(outt) -> omega_mech/1, Abs/1, Sign1/1
  Sign1/1 -> Product4/2
  Sum5/1 -> Product4/1
  Product11/1 -> integrator1/2(in)

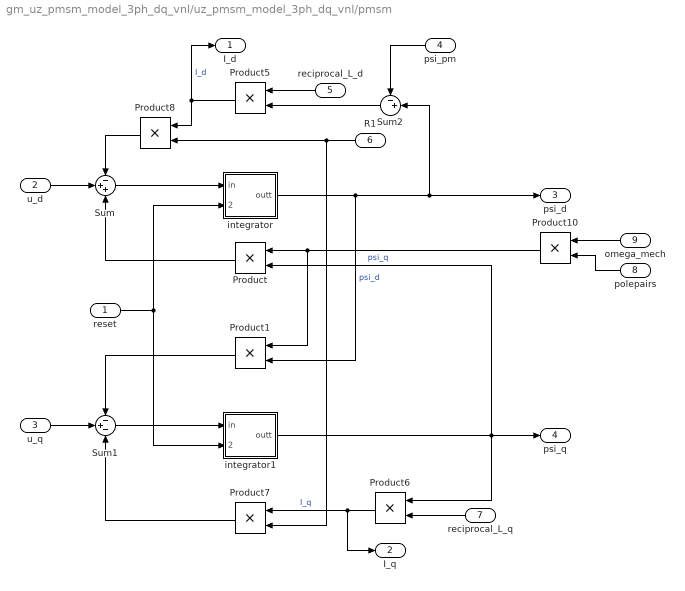
== system gm_uz_pmsm_model_3ph_dq_vnl/uz_pmsm_model_3ph_dq_vnl/pmsm ==
  reset : Inport
  u_d : Inport  Port=2
  u_q : Inport  Port=3
  psi_pm : Inport  Port=4
  reciprocal_L_d : Inport  Port=5
  R1 : Inport  Port=6
  reciprocal_L_q : Inport  Port=7
  polepairs : Inport  Port=8
  omega_mech : Inport  Port=9
  Product{,1,5..8,10} (7 alike) : Product
  Sum : Sum  Inputs=-++
  Sum1 : Sum  Inputs=-+-
  Sum2 : Sum  Inputs=-+|
  integrator : Subsystem
  integrator1 : Subsystem
  I_d : Outport
  I_q : Outport  Port=2
  psi_d : Outport  Port=3
  psi_q : Outport  Port=4
  wires:
  Sum1/1 -> integrator1/1(in)
  Product7/1 -> Sum1/3
  reciprocal_L_q/1 -> Product6/2
  polepairs/1 -> Product10/2
  Product8/1 -> Sum/1
  Sum2/1 -> Product5/2
  integrator/1(outt) -> Product1/2, Sum2/2, psi_d/1  "psi_d"
  Product10/1 -> Product/1, Product1/1
  Product6/1 -> Product7/1, I_q/1  "I_q"
  psi_pm/1 -> Sum2/1
  Sum/1 -> integrator/1(in)
  reset/1 -> integrator/2(reset), integrator1/2(reset)
  Product1/1 -> Sum1/1
  u_d/1 -> Sum/2
  integrator1/1(outt) -> psi_q/1, Product/2, Product6/1  "psi_q"
  reciprocal_L_d/1 -> Product5/1
  R1/1 -> Product8/2, Product7/2
  Product5/1 -> Product8/1, I_d/1  "I_d"
  Product/1 -> Sum/3
  u_q/1 -> Sum1/2
  omega_mech/1 -> Product10/1

== system gm_uz_pmsm_model_3ph_dq_vnl/uz_pmsm_model_3ph_dq_vnl/torque_calculation ==
  I_d : Inport
  I_q : Inport  Port=2
  psi_d : Inport  Port=3
  psi_q : Inport  Port=4
  polepairs : Inport  Port=5
  Factor : Gain  Gain=(3/2)
  Product2 : Product
  Product3 : Product
  Product9 : Product
  Sum3 : Sum  Inputs=-|+
  M_Mi : Outport
  wires:
  Factor/1 -> Product9/1  "M_Mi"
  polepairs/1 -> Product9/2
  Product9/1 -> M_Mi/1  "M_Mi"
  I_q/1 -> Product3/2
  I_d/1 -> Product2/1
  psi_d/1 -> Product3/1
  psi_q/1 -> Product2/2
  Product2/1 -> Sum3/1
  Product3/1 -> Sum3/2
  Sum3/1 -> Factor/1

== system gm_uz_pmsm_model_3ph_dq_vnl/Compare/Assert_outputs/RelErrCheck ==
  In1 : Inport
  In2 : Inport  Port=2
  "RelativeErrorCheck " : MATLAB Function  TreatAsAtomicUnit=on
  Out1 : Outport  VectorParamsAs1DForOutWhenUnconnected=off
  wires:
  "RelativeErrorCheck "/1(y) -> Out1/1
  In1/1 -> "RelativeErrorCheck "/1(P)
  In2/1 -> "RelativeErrorCheck "/2(R)

== system gm_uz_pmsm_model_3ph_dq_vnl/Compare/Assert_voltage_input_dq_out_axi_fb/RelErrCheck ==
  In1 : Inport
  In2 : Inport  Port=2
  "RelativeErrorCheck " : MATLAB Function  TreatAsAtomicUnit=on
  Out1 : Outport  VectorParamsAs1DForOutWhenUnconnected=off
  wires:
  "RelativeErrorCheck "/1(y) -> Out1/1
  In1/1 -> "RelativeErrorCheck "/1(P)
  In2/1 -> "RelativeErrorCheck "/2(R)

== system gm_uz_pmsm_model_3ph_dq_vnl/uz_pmsm_model_3ph_dq_vnl/mechanical_system/integrator1 ==
  reset : Inport
  in : Inport  Port=2
  Delay1 : Delay  DelayLength=1  ExternalReset=Level
      settings: InputPortMap=u0,r5
  Gain : Gain  Gain=ts  OutDataTypeStr=double
  Sum3 : Sum  Inputs=|++  OutDataTypeStr=double
  outt : Outport
  wires:
  Delay1/1 -> outt/1, Sum3/2
  Sum3/1 -> Delay1/1
  reset/1 -> Delay1/2
  Gain/1 -> Sum3/1
  in/1 -> Gain/1

== system gm_uz_pmsm_model_3ph_dq_vnl/uz_pmsm_model_3ph_dq_vnl/pmsm/integrator ==
  in : Inport
  reset : Inport  Port=2
  Delay1 : Delay  DelayLength=1  ExternalReset=Level
      settings: InputPortMap=u0,r5
  Gain : Gain  Gain=ts  OutDataTypeStr=double
  Sum3 : Sum  Inputs=|++  OutDataTypeStr=double
  outt : Outport
  wires:
  Sum3/1 -> Delay1/1
  Delay1/1 -> Sum3/2, outt/1
  in/1 -> Gain/1
  Gain/1 -> Sum3/1
  reset/1 -> Delay1/2

== system gm_uz_pmsm_model_3ph_dq_vnl/uz_pmsm_model_3ph_dq_vnl/pmsm/integrator1 ==
  in : Inport
  reset : Inport  Port=2
  Delay1 : Delay  DelayLength=1  ExternalReset=Level
      settings: InputPortMap=u0,r5
  Gain : Gain  Gain=ts  OutDataTypeStr=double
  Sum3 : Sum  Inputs=|++  OutDataTypeStr=double
  outt : Outport
  wires:
  Sum3/1 -> Delay1/1
  Delay1/1 -> outt/1, Sum3/2
  reset/1 -> Delay1/2
  Gain/1 -> Sum3/1
  in/1 -> Gain/1

== matlab function gm_uz_pmsm_model_3ph_dq_vnl/Compare/Assert_outputs/RelErrCheck/RelativeErrorCheck  ==
  data: P input; y output; R input; ToleranceValue parameter double
% Check if the relative error of R with respect to P is below
% ToleranceValue
% P, R are floating-point
function y = relErrCheck(P,R, ToleranceValue)
    tol = ToleranceValue;
    sz = numel(P);
    assert(sz == numel(R), 'Inputs P and R have different sizes.');
    y = false(1, sz);

    for ii=1:sz
        if (isnan(P(ii)) || isnan(R(ii)))
            if (isnan(P(ii)) && isnan(R(ii)))
                y(ii) = true;
            end
        elseif (isinf(P(ii)) || isinf(R(ii)))
            y(ii) = (P(ii) == R(ii));
        elseif (P(ii) == 0)
            y(ii) = (R(ii) == 0);
        else
            absdiff = abs(P(ii) - R(ii));
            relerr = absdiff/abs(P(ii));
            y(ii) = (relerr <= tol);
        end
    end
end

== matlab function gm_uz_pmsm_model_3ph_dq_vnl/Compare/Assert_voltage_input_dq_out_axi_fb/RelErrCheck/RelativeErrorCheck  ==
  data: P input; y output; R input; ToleranceValue parameter double
% Check if the relative error of R with respect to P is below
% ToleranceValue
% P, R are floating-point
function y = relErrCheck(P,R, ToleranceValue)
    tol = ToleranceValue;
    sz = numel(P);
    assert(sz == numel(R), 'Inputs P and R have different sizes.');
    y = false(1, sz);

    for ii=1:sz
        if (isnan(P(ii)) || isnan(R(ii)))
            if (isnan(P(ii)) && isnan(R(ii)))
                y(ii) = true;
            end
        elseif (isinf(P(ii)) || isinf(R(ii)))
            y(ii) = (P(ii) == R(ii));
        elseif (P(ii) == 0)
            y(ii) = (R(ii) == 0);
        else
            absdiff = abs(P(ii) - R(ii));
            relerr = absdiff/abs(P(ii));
            y(ii) = (relerr <= tol);
        end
    end
end
